simulink model "hexarotor"  (R2024a)
settings: configuration reference "standardSILConfiguraitonParams" (kept outside this file)
settings Model: Creator=jerem  LastModifiedBy=jerem
settings ConfigSetRef: SourceName=standardSILConfiguraitonParams  SourceLocation=Base Workspace

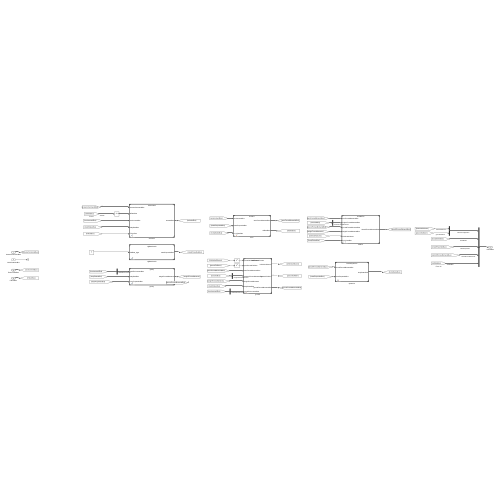
[thumbnail: Simulink's stored preview of the top-level diagram]
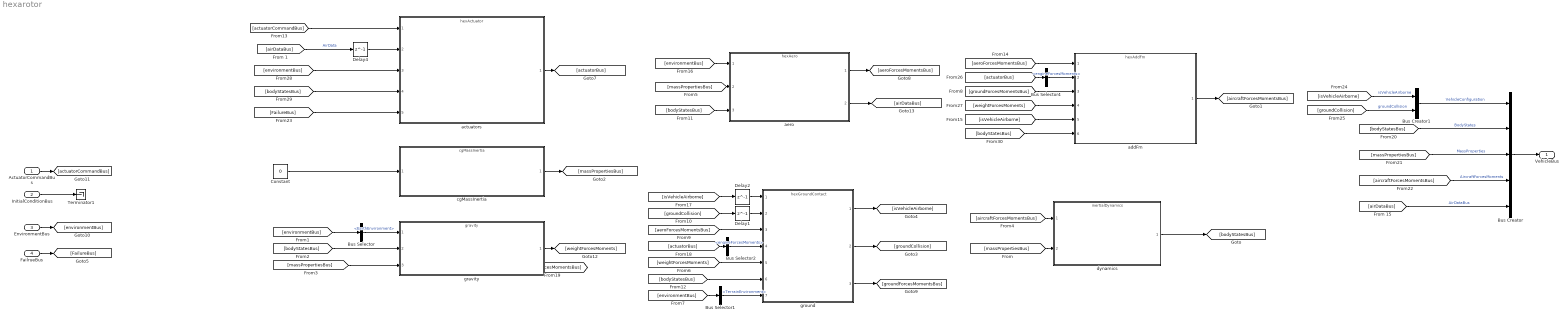
== system hexarotor ==
  ActuatorCommandBus : Inport  OutDataTypeStr=Bus: ActuatorCommandBus
  InitialConditionBus : Inport  Port=2
  EnvironmentBus : Inport  Port=3  OutDataTypeStr=Bus: EnvironmentBus
  FailrueBus : Inport  Port=4  OutDataTypeStr=Bus: FailureBus
  Bus Creator : BusCreator  Inputs=5  OutDataTypeStr=Bus: VehicleBus
  Bus Creator1 : BusCreator  Inputs=2  OutDataTypeStr=Bus: VehicleConfigurationBus
  Bus Selector : BusSelector  OutputSignals=EarthEnvironment
  Bus Selector1 : BusSelector  OutputSignals=TerrainEnvironment
  Bus Selector2 : BusSelector  OutputSignals=PropulsionBus.engineForcesMoments
  Bus Selector4 : BusSelector  OutputSignals=PropulsionBus.engineForcesMoments
  Constant : Constant  Value=0
  Delay1 : Delay  DelayLength=1  InitialCondition=0
  Delay2 : Delay  DelayLength=1  InitialCondition=0
  Delay4 : Delay  DelayLength=1  InitialCondition=0
  Terminator1 : Terminator
  actuators : ModelReference  ModelNameDialog=hexActuator.slx  SimulationMode=Normal  ModelReferenceVersion=1.33
  addFm : ModelReference  ModelNameDialog=hexAddFm.slx  SimulationMode=Normal  ModelReferenceVersion=1.2
  aero : ModelReference  ModelNameDialog=hexAero.slx  SimulationMode=Normal  ModelReferenceVersion=1.15
  cgMassInertia : ModelReference  ModelNameDialog=cgMassInertia.slx  SimulationMode=Normal  ModelReferenceVersion=1.42
  dynamics : ModelReference  ModelNameDialog=inertialDynamics.slx  SimulationMode=Normal  ModelReferenceVersion=1.34
  gravity : ModelReference  ModelNameDialog=gravity.slx  SimulationMode=Normal  ModelReferenceVersion=1.26
  ground : ModelReference  ModelNameDialog=hexGroundContact.slx  SimulationMode=Normal  ModelReferenceVersion=1.39
  VehicleBus : Outport  OutDataTypeStr=Bus: VehicleBus
  wires:
  [groundCollision] -> Bus Creator1/2  "groundCollision"
  Bus Creator1/1 -> Bus Creator/1  "VehicleConfiguration"
  [isVehicleAirborne] -> Bus Creator1/1  "isVehicleAirborne"
  [massPropertiesBus] -> Bus Creator/3  "MassProperties"
  [aircraftForcesMomentsBus] -> Bus Creator/4  "AircraftForcesMoments"
  [bodyStatesBus] -> Bus Creator/2  "BodyStates"
  Bus Creator/1 -> VehicleBus/1
  [airDataBus] -> Bus Creator/5  "AirDataBus"
  dynamics/1 -> [bodyStatesBus]
  [aircraftForcesMomentsBus] -> dynamics/1
  addFm/1 -> [aircraftForcesMomentsBus]
  cgMassInertia/1 -> [massPropertiesBus]
  [massPropertiesBus] -> dynamics/2
  InitialConditionBus/1 -> Terminator1/1
  ActuatorCommandBus/1 -> [actuatorCommandBus]
  EnvironmentBus/1 -> [environmentBus]
  [environmentBus] -> Bus Selector/1
  Bus Selector/1 -> gravity/1  "<EarthEnvironment>"
  [bodyStatesBus] -> gravity/2
  [massPropertiesBus] -> gravity/3
  gravity/1 -> [weightForcesMoments]
  Constant/1 -> cgMassInertia/1
  Delay4/1 -> actuators/2
  [bodyStatesBus] -> actuators/4
  [environmentBus] -> actuators/3
  [actuatorCommandBus] -> actuators/1
  [airDataBus] -> Delay4/1  "AirData"
  actuators/1 -> [actuatorBus]
  [bodyStatesBus] -> aero/3
  [massPropertiesBus] -> aero/2
  [environmentBus] -> aero/1
  [aeroForcesMomentsBus] -> addFm/1
  [actuatorBus] -> Bus Selector4/1
  [groundForcesMomentsBus] -> addFm/3
  [weightForcesMoments] -> addFm/4
  [isVehicleAirborne] -> addFm/5
  [bodyStatesBus] -> addFm/6
  ground/2 -> [groundCollision]
  ground/1 -> [isVehicleAirborne]
  ground/3 -> [groundForcesMomentsBus]
  Bus Selector2/1 -> ground/4  "<engineForcesMoments>"
  [environmentBus] -> Bus Selector1/1
  [weightForcesMoments] -> ground/5
  [aeroForcesMomentsBus] -> ground/3
  Delay2/1 -> ground/1
  [actuatorBus] -> Bus Selector2/1
  [groundCollision] -> Delay1/1
  [isVehicleAirborne] -> Delay2/1
  [bodyStatesBus] -> ground/6
  Delay1/1 -> ground/2
  Bus Selector1/1 -> ground/7  "<TerrainEnvironment>"
  aero/2 -> [airDataBus]
  aero/1 -> [aeroForcesMomentsBus]
  Bus Selector4/1 -> addFm/2  "<engineForcesMoments>"
  FailrueBus/1 -> [FailureBus]
  [FailureBus] -> actuators/5
